simulink model "finalMPC_FUNKAR"  (R2019b)
settings: Solver=VariableStepAuto  StartTime=0.0  StopTime=10.0  RelTol=1e-3
settings Model: Creator=Daniel  LastModifiedBy=trulsmartinsson

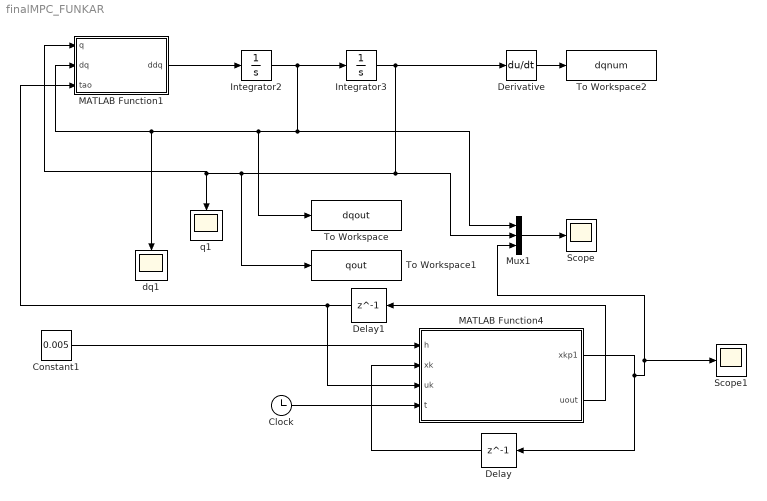
== system finalMPC_FUNKAR ==
  Clock : Clock
  Constant1 : Constant  Value=0.005
  Delay : Delay  DelayLength=1  InitialCondition=[0;pi+0.3;0.3;0.3]  SampleTime=0.005
  Delay1 : Delay  DelayLength=1  InitialCondition=[0;pi+0.3;0.3;0.3]  SampleTime=0.005
  Derivative : Derivative
  Integrator2 : Integrator  InitialCondition=[0;0]
  Integrator3 : Integrator  InitialCondition=[0;pi+0.1]
  MATLAB Function1 : MATLAB Function  TreatAsAtomicUnit=on  SystemSampleTime=0.001
  MATLAB Function4 : MATLAB Function  TreatAsAtomicUnit=on  SystemSampleTime=0.005
  Mux1 : Mux  Inputs=3
  Scope : Scope
  Scope1 : Scope
  To Workspace : ToWorkspace  VariableName=dqout  SaveFormat=Timeseries  SampleTime=-1
  To Workspace1 : ToWorkspace  VariableName=qout  SampleTime=-1
  To Workspace2 : ToWorkspace  VariableName=dqnum  SaveFormat=Timeseries  SampleTime=-1
  dq1 : Scope
  q1 : Scope
  wires:
  Integrator3/1 -> Derivative/1, Mux1/2, To Workspace1/1, MATLAB Function1/1(q), q1/1
  Integrator2/1 -> Mux1/1, To Workspace/1, MATLAB Function1/2(dq), dq1/1, Integrator3/1
  Constant1/1 -> MATLAB Function4/1(h)
  MATLAB Function1/1(ddq) -> Integrator2/1
  MATLAB Function4/1(xkp1) -> Delay/1, Mux1/3, Scope1/1
  Delay/1 -> MATLAB Function4/2(xk)
  Mux1/1 -> Scope/1
  Clock/1 -> MATLAB Function4/4(t)
  Derivative/1 -> To Workspace2/1
  MATLAB Function4/2(uout) -> Delay1/1
  Delay1/1 -> MATLAB Function1/3(tao), MATLAB Function4/3(uk)

== matlab function finalMPC_FUNKAR/MATLAB Function1 ==
  data: q input; ddq output; dq input; tao input
function  ddq  = testing(q,dq,tao)
%% q= [phi, theta],   dq = [dphi, dtheta]
%tao2=[0;tao];
%tao2 = [tao;0]; - DENNA FUNKADE TIDIGARE
tao2 = [tao(1);0];
phi = q(1,1);
theta = q(2,1);
dphi = dq(1,1);
dtheta = dq(2,1);
%Given parameters - "competition.pdf"
la  = 75*10^-3;       %[m]      - Length of arm
r  = 43*10^-3;       %[m]      - Base radius
lp  = 31.5*10^-3;     %[m]      - Length of pendulum
J  = 125*10^-6;      %[kgm^2]  - Base moment of inertia
g  = 9.8;            %[m/s^2]  - Gravity
Jc = 2.55*10^-6;     %[kgm^2]  - Moment of inertia of pendulum around c.o.m
M  = 5.44*10^-3;     %[kg]     - Mass of pendulum point mass
Jp = 7.95*10^-6;     %[kgm^2]  - Moment of inertia of pend around pivot

%Still unknown - Try to guess these as a first step
ma = 10*10^-3;       %[kg] - Mass of arm       - Try 10g
mp = 5*10^-3;        %[kg] - Mass of pendulum  - Try 5g

%Equation (17)
alpha   = J + (M + (1/3)*ma + mp)*la^2;
beta    = (M + (1/3)*mp)*lp^2;
gamma   = (M + (1/2)*mp)*la*lp;
delta   = (M + (1/2)*mp)*g*lp;

D = [(alpha + beta*sin(theta)^2),(gamma*cos(theta));(gamma*cos(theta)),(beta)];
C = [(beta*cos(theta)*sin(theta)*dtheta),(beta*cos(theta)*sin(theta)*dphi - gamma*sin(theta)*dtheta);(-beta*cos(theta)*sin(theta)*dphi),(0)];
G = [0;-delta*sin(theta)];

% ddq = inv(D)*(tao2 - C*dq - G);
ddq = D\(tao2 - C*dq - G);
end

== matlab function finalMPC_FUNKAR/MATLAB Function4 ==
  data: h input; xkp1 output; xk input; uk input; t input; uout output
function [xkp1, uout] = MPC(h,xk,uk,t) 
coder.extrinsic('plot')
coder.extrinsic('spy')
coder.extrinsic('quadprog')
coder.extrinsic('legend')
coder.extrinsic('kron')
coder.extrinsic('repmat')
coder.extrinsic('optimoptions')

persistent xbar;

%Given parameters - "competition.pdf"

la  = 75*10^-3;       %[m]      - Length of arm
r  = 43*10^-3;       %[m]      - Base radius
lp  = 31.5*10^-3;     %[m]      - Length of pendulum
J  = 125*10^-6;      %[kgm^2]  - Base moment of inertia
g  = 9.8;            %[m/s^2]  - Gravity
Jc = 2.55*10^-6;     %[kgm^2]  - Moment of inertia of pendulum around c.o.m
M  = 5.44*10^-3;     %[kg]     - Mass of pendulum point mass
Jp = 7.95*10^-6; 

%Still unknown - Try to guess these as a first step
ma = 10*10^-3;       %[kg] - Mass of arm       - Try 10g
mp = 5*10^-3;        %[kg] - Mass of pendulum  - Try 5g

%Equation (17)
alpha   = J + (M + (1/3)*ma + mp)*la^2;
beta    = (M + (1/3)*mp)*lp^2;
gamma   = (M + (1/2)*mp)*la*lp;
delta   = (M + (1/2)*mp)*g*lp;

Hp = 100;
% uk=[uk];
% Hu = 15+1;
% xbar = zeros(4*Hp,1);
% xbar(1:4) = xk;
% ubar = repmat([0;0;1],Hu,1);
% ubar(1:2) = uk;
% 
% Ahp=zeros(4*Hp,4*Hp);
% Bhp=zeros(4*Hp,3*Hp);

% xbarref = repmat([0;pi;0;0;0], [Hp,1]);
xbarrefx = repmat([0;pi;0;0], [Hp,1]);
xbarrefu = zeros(Hp,1);
xbarrefu(1:4) = uk;
xbarref = [xbarrefx;xbarrefu];


Nx = 4;
if isempty(xbar)
    xbar = zeros((Nx+1)*Hp,1);
    xbar = xbarref;
end
xbar = xbarref;

[Aeq, Beq] = computeAeqBeq(Hp,xbar,xk,alpha,beta,gamma,delta,h);

xbar0 = zeros((Nx+1)*Hp,1);
xtraj = zeros(Hp,Nx);
Xbaropt = zeros((Nx+1)*Hp,1);
% Xbaropt = fmincon(@cost,xbar0,[],[],Aeq,Beq);

LB = -1000*ones(Hp*(Nx+1),1);
UB = +1000*ones(Hp*(Nx+1),1);
Hx = kron(eye(Hp-1),diag([1/pi^2,1/pi^2,1/3^2,1/3^2]));
Hf = 10*diag([1/pi^2,1/pi^2,1/3^2,1/3^2]);
Hu = (1/0.2^2)*eye(Hp);
H = blkdiag(Hx,Hf,Hu);
f = -1*xbarref'*H;
opt = optimoptions('quadprog'); 
newopt = optimoptions(opt, 'ConstraintTolerance', 1e-12, 'OptimalityTolerance', 1e-12, 'MaxIterations', 1e3)

Xbaropt = quadprog(H,f',[],[],Aeq,Beq,LB,UB,xbar,newopt);
xtraj = reshape(Xbaropt(1:Nx*Hp), [Nx,Hp])';
xref = reshape(xbarref(1:Nx*Hp), [Nx,Hp])';
subplot(1,3,1)
cla;
plot(xtraj(:,1:2));
hold on;
plot(xref);
legend('phi', 'theta');
subplot(1,3,2);
cla;
plot(xtraj(:,3:4));
hold on
plot(diff(xtraj(:,1:2) ,1)/h)
legend( 'dphi', 'dtheta');
subplot(1,3,3)
plot(Xbaropt(Nx*Hp+1:end))




xbar = Xbaropt;

disp(t)
if t > 4
    a = 1;
end

uout = Xbaropt(Nx*Hp+1);  %DENNA FUNKADE TIDIGARE



[Ad,Bd,Gd]=linAndDis(xk,uout,alpha,beta,gamma,delta,h);
xkp1=Ad*xk + Bd*uout+ Gd;

% for i = 2:2
%     theta=xbar((i-1)*4-2,1);
%     dphi=xbar((i-1)*4-1,1);
%     dtheta=xbar((i-1)*4,1);  
% D = [(alpha + beta*sin(theta)^2),(gamma*cos(theta));(gamma*cos(theta)),(beta)];
% C = [(beta*cos(theta)*sin(theta)*dtheta),(beta*cos(theta)*sin(theta)*dphi - gamma*sin(theta)*dtheta);(-beta*cos(theta)*sin(theta)*dphi),(0)];
% G = [0;-delta*sin(theta)];
% f_x = D\(-C -G/xbar((i-1)*4-1:(i-1)*4));
% f_u = D\[1;1];
% 
% V1 = xk(1:2)-diag(xbar((i-1)*4-1:(i-1)*4))*xbar((i-1)*4-3:(i-1)*4-2);
% A1 = diag(xbar((i-1)*4-1:(i-1)*4));
% B1 = zeros(2,2);
% V2 = xbar((i-1)*4-1:(i-1)*4)-f_x*xbar((i-1)*4-3:(i-1)*4-2)-diag(f_u)*ubar(1:2);
% A2 = f_x;
% B2= diag(f_u);
% Hd =ss([A1,[0,0;0,0];[0,0;0,0],A2],[B1,V1;B2,V2],[0,0,0,0],[],h);
% Ad = Hd.A;
% Bd = Hd.B;
% Ahp(4*i-3:4*i, 4*i-3:4*i)= Ad;
% Bhp(4*i-3:4*i, 3*i-2:3*i) = Bd;
% 
%     xbar((i*4-3):(i*4)) = xbar((i-1)*4-3:(i-1)*4) + h*(Ad*xbar((i-1)*4-3:(i-1)*4) + Bd*ubar((i-1)*3-2:(i-1)*3));
% end
end
function [f,jacFx,jacFu] = evalFun(x,u,alpha,beta,gamma,delta)
tau=u;
theta=x(2,1);
dphi=x(3,1);
dtheta=x(4,1);
dq=x(3:4);
D = [(alpha + beta*sin(theta)^2),(gamma*cos(theta));(gamma*cos(theta)),(beta)];
C = [(beta*cos(theta)*sin(theta)*dtheta),(beta*cos(theta)*sin(theta)*dphi - gamma*sin(theta)*dtheta);(-beta*cos(theta)*sin(theta)*dphi),(0)];
G = [0;-delta*sin(theta)];

jacFx = [ 0,                                                                                                                                                                                                                                                                                                                                                                                                                                                                                                                                                                                                                                                                                                                                                                                                                                                 0,                                                                                                                                                                                         1,                                                                                                                                               0;
0,                                                                                                                                                                                                                                                                                                                                                                                                                                                                                                                                                                                                                                                                                                                                                                                                                                                 0,                                                                                                                                                                                         0,                                                                                                                                               1;
0,                                                                                                                                                                                                                               (delta*gamma*sin(theta)^2 - delta*gamma*cos(theta)^2 - 2*beta^2*dphi*dtheta*cos(theta)^2 - beta*dphi^2*gamma*cos(theta)^3 + 2*beta^2*dphi*dtheta*sin(theta)^2 + beta*dtheta^2*gamma*cos(theta) + 2*beta*dphi^2*gamma*cos(theta)*sin(theta)^2)/(alpha*beta - gamma^2*cos(theta)^2 + beta^2*sin(theta)^2) + ((2*cos(theta)*sin(theta)*beta^2 + 2*cos(theta)*sin(theta)*gamma^2)*(delta*gamma*cos(theta)*sin(theta) - beta*dtheta^2*gamma*sin(theta) - beta*tau + beta*dphi^2*gamma*cos(theta)^2*sin(theta) + 2*beta^2*dphi*dtheta*cos(theta)*sin(theta)))/(alpha*beta - gamma^2*cos(theta)^2 + beta^2*sin(theta)^2)^2,                                            -(2*beta^2*dtheta*cos(theta)*sin(theta) + 2*beta*dphi*gamma*cos(theta)^2*sin(theta))/(alpha*beta - gamma^2*cos(theta)^2 + beta^2*sin(theta)^2),               -(2*dphi*cos(theta)*sin(theta)*beta^2 - 2*dtheta*gamma*sin(theta)*beta)/(alpha*beta - gamma^2*cos(theta)^2 + beta^2*sin(theta)^2);
0, (gamma*tau*sin(theta) - dtheta^2*gamma^2*cos(theta)^2 - beta^2*dphi^2*sin(theta)^4 + dtheta^2*gamma^2*sin(theta)^2 + alpha*delta*cos(theta) + alpha*beta*dphi^2*cos(theta)^2 - alpha*beta*dphi^2*sin(theta)^2 + 3*beta*delta*cos(theta)*sin(theta)^2 + 3*beta^2*dphi^2*cos(theta)^2*sin(theta)^2 + 2*beta*dphi*dtheta*gamma*cos(theta)^3 - 4*beta*dphi*dtheta*gamma*cos(theta)*sin(theta)^2)/(alpha*beta - gamma^2*cos(theta)^2 + beta^2*sin(theta)^2) - ((2*cos(theta)*sin(theta)*beta^2 + 2*cos(theta)*sin(theta)*gamma^2)*(alpha*delta*sin(theta) - gamma*tau*cos(theta) + beta*delta*sin(theta)^3 + beta^2*dphi^2*cos(theta)*sin(theta)^3 - dtheta^2*gamma^2*cos(theta)*sin(theta) + alpha*beta*dphi^2*cos(theta)*sin(theta) + 2*beta*dphi*dtheta*gamma*cos(theta)^2*sin(theta)))/(alpha*beta - gamma^2*cos(theta)^2 + beta^2*sin(theta)^2)^2, (2*beta^2*dphi*cos(theta)*sin(theta)^3 + 2*alpha*beta*dphi*cos(theta)*sin(theta) + 2*beta*dtheta*gamma*cos(theta)^2*sin(theta))/(alpha*beta - gamma^2*cos(theta)^2 + beta^2*sin(theta)^2), -(2*dtheta*gamma^2*cos(theta)*sin(theta) - 2*beta*dphi*gamma*cos(theta)^2*sin(theta))/(alpha*beta - gamma^2*cos(theta)^2 + beta^2*sin(theta)^2)];
 
jacFu =  [                                                                            0;
                                                                             0;
                beta/(alpha*beta - gamma^2*cos(theta)^2 + beta^2*sin(theta)^2);
 -(gamma*cos(theta))/(alpha*beta - gamma^2*cos(theta)^2 + beta^2*sin(theta)^2)];
f = [dq;D\([tau;0] - C * dq - G) ];

end

function [Ad,Bd,Gd]=linAndDis(xk,uk,alpha,beta,gamma,delta,h)
[f,jacFx,jacFu]=evalFun(xk,uk,alpha,beta,gamma,delta);
% xdot= f+(jacFx*(x-xk)+jacFu*(u-uk));
% xdot=f-jacFx*xk-jacFu*uk + jacFx*x+ jacFu*u;
Gc=f-jacFx*xk-jacFu*uk;
Ac=jacFx;
Bc=jacFu;
Ace= Ac;
Bce=[Bc,Gc];
Md = expm(h*[Ace, Bce; zeros(2,6)]);
Ade=Md(1:4,1:4);
Bde=Md(1:4,5:6);
Ad=Ade;
Bd=Bde(:,1);
Gd=Bde(:,2);
% I = eye(2);
% z = zeros(2,2);
% Ad=[I,h*I;z,I];
% Bd = [h^2/2*ones(2,1);h*ones(2,1)];
% Gd = zeros(4,1);
end

function [Aeq, Beq] = computeAeqBeq(Hp,xbar,xk,alpha,beta,gamma,delta,h)
coder.extrinsic('spy')
I14 = 1:4;
Nx  = 4;
Aeq = zeros(Hp*Nx, (Nx+1)*Hp);
Beq = zeros(Hp*Nx, 1);
for i = 0:(Hp-2)
    if i < Hp-2
        xi = xbar(I14+Nx+Nx*i);
        ui = xbar(Hp*Nx+1+i);
    else
        xi = xbar(I14+Nx*i);
        ui = xbar(Hp*Nx+i);
    end
    if i == 0
        xi = xk;
        ui = xbar(Hp*Nx+2);
    end
     
    xi = xk;
    ui = xbar(Nx*Hp+2);
    [Ad,Bd,Gd]=linAndDis(xi, ui,alpha,beta,gamma,delta,h);
    Aeq(Nx*i+I14, Nx*i+I14)     = Ad;
    Aeq(Nx*i+I14, Nx*(i+1)+I14) = -eye(Nx);   
    Aeq(Nx*i+I14, Nx*Hp+i+1)      = Bd;
    Beq(Nx*i+I14, 1)            = - Gd;
%     spy(Aeq);
end
Aeq(end-3:end, I14) = eye(4);
Beq(end-3:end, 1) = xk;

% subplot(1,2,1); 
% subplot(1,2,2); 
% spy(Beq);

end
